simulink model "square_model"  (R2016b)
settings: Solver=VariableStepAuto  StartTime=0.0  StopTime=60  RelTol=1e-3
values from neighbouring files (symbols this model uses):
  coef_a = 1    [MRAC_test.m]    (also in model_gen.m)
  coef_b = 2*zta*w_n    [MRAC_test.m]    (also in model_gen.m)
  coef_c = w_n^2    [MRAC_test.m]    (also in model_gen.m = w_n)
  numer = coef_c    [model_gen.m]
  pitch_mpu_madgwick = 1    [model_gen.m]
  throt = 1.5    [model_gen.m]
libraries: simulink x2
settings Model: Creator=CFreeman  LastModifiedBy=CFreeman

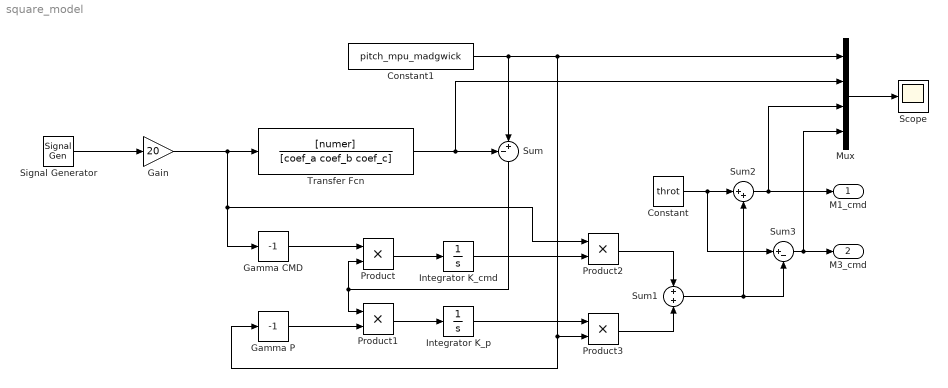
== system square_model ==
  Constant : Constant  Value=throt
  Constant1 : Constant  Value=pitch_mpu_madgwick
  Gain : Gain  Gain=20
  Gamma CMD : simulink/Math Operations/Slider Gain  low=-10  gain=-1  high=-1
  Gamma P : simulink/Math Operations/Slider Gain  low=-10  gain=-1  high=-1
  Integrator K_cmd : Integrator
  Integrator K_p : Integrator
  Mux : Mux
  Product{,1..3} (4 alike) : Product
  Scope : Scope
  Signal Generator : SignalGenerator  Units=rad/sec
  Sum : Sum  Inputs=-+|
  Sum1 : Sum
  Sum2 : Sum  Inputs=|++
  Sum3 : Sum  Inputs=|+-
  Transfer Fcn : TransferFcn  Numerator=[numer]  Denominator=[coef_a coef_b coef_c]
  M1_cmd : Outport
  M3_cmd : Outport  Port=2
  wires:
  Signal Generator/1 -> Gain/1
  Gain/1 -> Product2/1, Gamma CMD/1, Transfer Fcn/1
  Transfer Fcn/1 -> Mux/2, Sum/1
  Gamma CMD/1 -> Product/1
  Gamma P/1 -> Product1/2
  Product/1 -> Integrator K_cmd/1
  Integrator K_cmd/1 -> Product2/2
  Product2/1 -> Sum1/1
  Product1/1 -> Integrator K_p/1
  Product3/1 -> Sum1/2
  Integrator K_p/1 -> Product3/1
  Constant/1 -> Sum3/1, Sum2/1
  Sum1/1 -> Sum3/2, Sum2/2
  Sum3/1 -> Mux/4, M3_cmd/1
  Sum2/1 -> Mux/3, M1_cmd/1
  Constant1/1 -> Sum/2, Product3/2, Gamma P/1, Mux/1
  Sum/1 -> Product1/1, Product/2
  Mux/1 -> Scope/1
